simulink library "srx_platform"  (Simulink 8.2)
settings: Solver=ode1  StartTime=0.0  StopTime=Inf  FixedStep=0.001  RelTol=1e-3
PostLoadFcn:
  | , if any(exist('dsrtsu_mdlpostloadfcn', 'file') == [2, 3, 6]), try dsrtsu_mdlpostloadfcn('Execute', bdroot); catch fprintf('Error in PostLoadFcn (dsrtsu_mdlpostloadfcn) for model "%s":\n %s\n', bdroot, lasterr); end, end,
libraries: rtican x23, rtiethernetudplib x4, srx_initialize x4, rtiflashlib x2, topr5_adapter x1
(part 2 of 6)

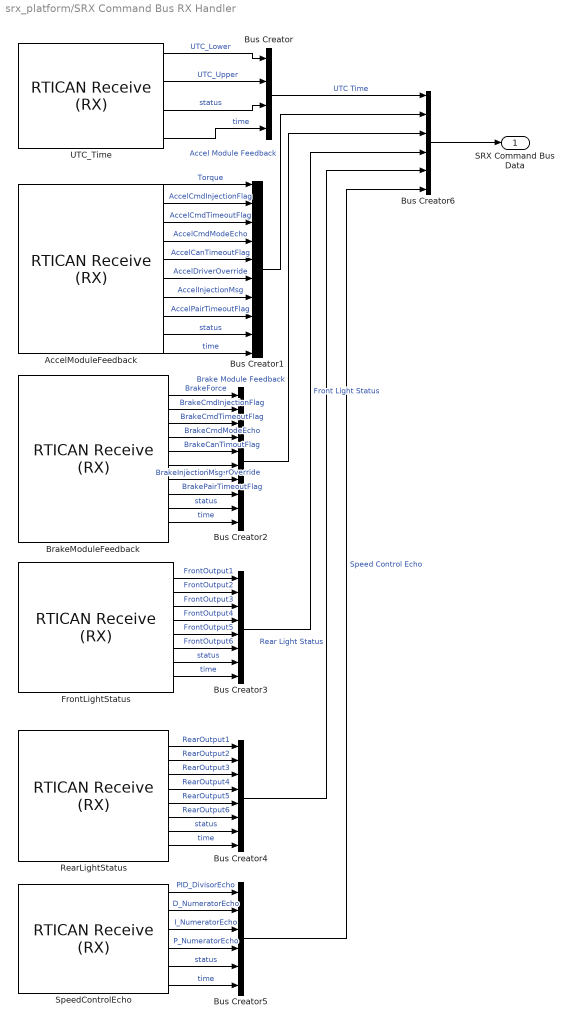
== system srx_platform/SRX Command Bus RX Handler ==
  AccelModuleFeedback : rtican/RTICAN Receive (RX)   Reserved1=[]  Reserved2=[]  Reserved3=[]  Reserved4=[]  SfcnMessage=[]  Msg_Struct=[]  BoardTypeNo=[]  BoardNo=[]  ChannelNo=[]  Parameters=[]  DialogFcn=[]  UnitName=[]  Revision=[]  UnitValues=[]  DSProperties=struct('RTI',struct('Version',uint32(5),'BlockType',struct('isSLSource',uint8(1),'isSLSink',uint8(1),'isHWSource',uint8(0),'isHWSink',uint8(0),'isSetup',uint8(0),'isInline',uint8(1),'isNonInline',uint8(0),'isInterrupt',uint8(0),'isChannelwise',uint8(0)),'IOBoardType','RTICAN','UnitType','MESSAGE','Identifier','RX','DialogType','MSVC','BlockSet','RTICAN','SlaveProcessor','CAN'))  RTIBlockInterface=struct('OutputPortsWidth',int32([1 1 1 1 1 1 1 1 1 1]),'OutputPortsActive',[1 1 1 1 1 1 1 1 1 1],'OutputPortsName',{{'Torque','AccelCmdInjectionFlag','AccelCmdTimeoutFlag','AccelCmdModeEcho','AccelCanTimeoutFlag','AccelDriverOverride','AccelInjectionMsg','AccelPairTimeoutFlag',['RX status'],['RX time']}},'OutputPortsDataType',{{'SS_UINT32','SS_BOOLEAN','SS_BOOLEAN','SS_UINT8','SS_BOOLEAN','SS_BOOLEAN','SS_BOOLEAN','SS_BOOLEAN','SS_DOUBLE','SS_DOUBLE'}},'OutputPortsLabel',{{'Torque','AccelCmdInjectionFlag','AccelCmdTimeoutFlag','AccelCmdModeEcho','AccelCanTimeoutFlag','AccelDriverOverride','AccelInjectionMsg','AccelPairTimeoutFlag','',''}},'OutputPortsLabelMode','ON','InputPortsWidth',int32(0),'InputPortsActive',0,'DialogFcn','rtican_message_interface_gui','BlockDisplay',{{'','center'}},'IconTransparency','on','ParameterTunableNames',{{}},'InitLevel',3,'BlockName',struct('Token',{{'AccelModuleFeedback'}}),'SampleTime',{{-1}},'TriggerPort',{{'none'}},'EnablePort',{{'none'}})  RTIBlockParameters=struct('BoardTypeNo',{{1,'OFF',[]}},'BoardNo',{{2,'ON',[1 16]}},'ChannelNo',{{1,'ON',[1 2]}},'Parameters',{{struct('DataFileSupport',struct('DataFileSelectedMaster',1,'DataFileSelectedLocal',1,'DataFileName','c:\users\leidos\development\carmaplatform\microautobox\src\data_files\srx_command.dbc|','DataFileDate',['17-Aug-2015 10:52:13'],'SelectedFile','..\data_files\srx_command.dbc','InterfaceFcn','rtican_dbc_file_parser'),'Options',struct('StatusSelected',1,'TimeSelected',1,'DeltaTimeSelected',0,'BytePortSelected',0,'MessageLengthSelected',0,'TriggerPort',struct('Selected',0,'TriggerType',0),'UserCoding',struct('Selected',0,'InterfaceFile','UserDecodingFile','FcnName','UserDecodeFcn','InportSelected',0,'InportWidth',1,'OutportSelected',0,'OutportWidth',1),'EnablePortSelected',0,'SignalOnPortnameSelected',1,'UseRXService',1),'Message',struct('MsgOnBlocknameSelected',1,'MsgName','AccelModuleFeedback','MsgIdFormat',0,'MsgId',416,'MsgLength',4,'NumSignals',8,'SampleTime',-1,'Signal',struct('SgnName',{'Torque','AccelCmdInjectionFlag','AccelCmdTimeoutFlag','AccelCmdModeEcho','AccelCanTimeoutFlag','AccelDriverOverride','AccelInjectionMsg','AccelPairTimeoutFlag'},'SgnStartBit',{0,24,25,26,28,29,30,31},'SgnLength',{24,1,1,2,1,1,1,1},'ByteLayout',{2,2,2,2,2,2,2,2},'Factor',{1,1,1,1,1,1,1,1},'Offset',{0,0,0,0,0,0,0,0},'SgnComment',{'','','','','','','',''},'SgnUnit',{'','','','','','','',''},'Min',{0,0,0,0,0,0,0,0},'Max',{0,0,0,0,0,0,0,0},'SgnType',{0,0,0,0,0,0,0,0},'SLDataType',{'SS_UINT32','SS_BOOLEAN','SS_BOOLEAN','SS_UINT8','SS_BOOLEAN','SS_BOOLEAN','SS_BOOLEAN','SS_BOOLEAN'},'DataType',{0,0,0,0,0,0,0,0},'ModeValue',{-1,-1,-1,-1,-1,-1,-1,-1}),'MsgIdNumFormat',0,'MsgComment',{{''}}),'Version',1.2,'general',struct('isFromLib',0)),'OFF',[]}},'GroupId',{{struct('Group',{{'RTICAN'}},'No',3,'Behavior',{{'NAMECHANGE'}},'BlockType',{{'SINK'}},'NameChangeFlag',0),'OFF',[]}},'SFcnRTICANMessage',{{struct('MsgType','RX','SFcnPortType','Scalar','MsgName','AccelModuleFeedback','MsgIdFormat','STD','MsgId',416,'MsgLength',4,'NumSignals',8,'SampleTime',-1,'Signal',struct('SgnName',{'Torque','AccelCmdInjectionFlag','AccelCmdTimeoutFlag','AccelCmdModeEcho','AccelCanTimeoutFlag','AccelDriverOverride','AccelInjectionMsg','AccelPairTimeoutFlag'},'SgnStartBit',{0,24,25,26,28,29,30,31},'SgnLength',{24,1,1,2,1,1,1,1},'ByteLayout',{['motorola back.'],['motorola back.'],['motorola back.'],['motorola back.'],['motorola back.'],['motorola back.'],['motorola back.'],['motorola back.']},'Factor',{1,1,1,1,1,1,1,1},'Offset',{0,0,0,0,0,0,0,0},'SgnType',{'standard','standard','standard','standard','standard','standard','standard','standard'},'SLDataType',{'SS_UINT32','SS_BOOLEAN','SS_BOOLEAN','SS_UINT8','SS_BOOLEAN','SS_BOOLEAN','SS_BOOLEAN','SS_BOOLEAN'},'DataType',{['unsigned int'],['unsigned int'],['unsigned int'],['unsigned int'],['unsigned int'],['unsigned int'],['unsigned int'],['unsigned int']},'ModeValue',{-1,-1,-1,-1,-1,-1,-1,-1}),'StatusSelected','yes','TimeSelected','yes','DeltaTimeSelected','no','BytePortSelected','no','MessageLengthSelected','no','TriggerPort',struct('Selected','no','TriggerType',0),'UserCoding',struct('Selected','no','InterfaceFile','UserDecodingFile','FcnName','UserDecodeFcn','InportSelected','no','InportWidth',1,'OutportSelected','no','OutportWidth',1),'EnablePortSelected','no','UseRXService','yes','BoardType','DS1','BoardNo',2,'ControllerNo',1),'OFF',[]}},'TLCFileName',{{'rtican_rx_message','OFF',[]}})  RTISFcnParameters=struct('SFcnRTICANMessage','struct','TLCFileName','char')  RTIBlockParaDefault=struct('BoardTypeNo',4302,'BoardNo',1,'ChannelNo',1,'Parameters',struct('DataFileSupport',struct('DataFileSelectedMaster',0,'DataFileSelectedLocal',0,'DataFileName','','DataFileDate','','SelectedFile',['<no file selected>']),'Options',struct('StatusSelected',1,'TimeSelected',1,'DeltaTimeSelected',1,'BytePortSelected',0,'MessageLengthSelected',0,'TriggerPort',struct('Selected',0,'TriggerType','rising'),'UserCoding',struct('Selected',0,'InterfaceFile','UserDecodingFile','FcnName','UserDecodeFcn','InportSelected',0,'InportWidth',1,'OutportSelected',0,'OutportWidth',1),'EnablePortSelected',0,'SignalOnPortnameSelected',1,'UseRXService',0),'Message',struct('MsgOnBlocknameSelected',0,'MsgName',['RX Message'],'MsgIdFormat',0,'MsgId',100,'MsgLength',8,'NumSignals',1,'SampleTime',-1,'Signal',struct('SgnName',['RX signal'],'SgnStartBit',0,'SgnLength',8,'SgnType',0,'ModeValue',-1,'DataType',0,'SLDataType','SS_DOUBLE','ByteLayout',0,'Factor',1,'Offset',0,'Min',0,'Max',255,'SgnComment',{{}},'SgnUnit',''),'MsgIdNumFormat',0,'MsgComment',{{''}}),'Version',1.2,'general',struct('isFromLib',1)),'GroupId',struct('Group',{{'RTICAN'}},'No',1,'Behavior',{{'NAMECHANGE'}},'BlockType',{{'SINK'}},'NameChangeFlag',0),'SFcnRTICANMessage',struct('MsgType','RX','MsgName',['RX Message'],'MsgIdFormat','STD','MsgId',100,'MsgLength',8,'NumSignals',1,'SampleTime',-1,'Signal',struct('SgnName',['RX signal'],'SgnStartBit',0,'SgnLength',8,'SgnType','standard','ModeValue',-1,'DataType',['unsigned int'],'ByteLayout',['little endian'],'SLDataType','SS_DOUBLE','Factor',1,'Offset',0),'StatusSelected','yes','TimeSelected','yes','DeltaTimeSelected','yes','BytePortSelected','no','MessageLengthSelected','no','EnablePortSelected','no','UserCoding',struct('Selected','no','InterfaceFile','UserDecodingFile','FcnName','UserDecodeFcn','InportSelected','no','InportWidth',1,'OutportSelected','no','OutportWidth',1),'TriggerPort',struct('Selected','no','TriggerType','rising'),'UseRXService','no','BoardType','DS4302','BoardNo',1,'ControllerNo',1,'SFcnPortType','Scalar'),'TLCFileName','rtican_rx_message')
      settings: AttributesFormatString=Group Id: RTICAN3\n
  BrakeModuleFeedback : rtican/RTICAN Receive (RX)   Reserved1=[]  Reserved2=[]  Reserved3=[]  Reserved4=[]  SfcnMessage=[]  Msg_Struct=[]  BoardTypeNo=[]  BoardNo=[]  ChannelNo=[]  Parameters=[]  DialogFcn=[]  UnitName=[]  Revision=[]  UnitValues=[]  DSProperties=struct('RTI',struct('Version',uint32(5),'BlockType',struct('isSLSource',uint8(1),'isSLSink',uint8(1),'isHWSource',uint8(0),'isHWSink',uint8(0),'isSetup',uint8(0),'isInline',uint8(1),'isNonInline',uint8(0),'isInterrupt',uint8(0),'isChannelwise',uint8(0)),'IOBoardType','RTICAN','UnitType','MESSAGE','Identifier','RX','DialogType','MSVC','BlockSet','RTICAN','SlaveProcessor','CAN'))  RTIBlockInterface=struct('OutputPortsWidth',int32([1 1 1 1 1 1 1 1 1 1]),'OutputPortsActive',[1 1 1 1 1 1 1 1 1 1],'OutputPortsName',{{'BrakeForce','BrakeCmdInjectionFlag','BrakeCmdTimeoutFlag','BrakeCmdModeEcho','BrakeCanTimoutFlag','BrakeDriverOverride','BrakeInjectionMsg','BrakePairTimeoutFlag',['RX status'],['RX time']}},'OutputPortsDataType',{{'SS_DOUBLE','SS_BOOLEAN','SS_BOOLEAN','SS_UINT8','SS_BOOLEAN','SS_BOOLEAN','SS_BOOLEAN','SS_BOOLEAN','SS_DOUBLE','SS_DOUBLE'}},'OutputPortsLabel',{{'BrakeForce','BrakeCmdInjectionFlag','BrakeCmdTimeoutFlag','BrakeCmdModeEcho','BrakeCanTimoutFlag','BrakeDriverOverride','BrakeInjectionMsg','BrakePairTimeoutFlag','',''}},'OutputPortsLabelMode','ON','InputPortsWidth',int32(0),'InputPortsActive',0,'DialogFcn','rtican_message_interface_gui','BlockDisplay',{{'','center'}},'IconTransparency','on','ParameterTunableNames',{{}},'InitLevel',3,'BlockName',struct('Token',{{'BrakeModuleFeedback'}}),'SampleTime',{{-1}},'TriggerPort',{{'none'}},'EnablePort',{{'none'}})  RTIBlockParameters=struct('BoardTypeNo',{{1,'OFF',[]}},'BoardNo',{{2,'ON',[1 16]}},'ChannelNo',{{1,'ON',[1 2]}},'Parameters',{{struct('DataFileSupport',struct('DataFileSelectedMaster',1,'DataFileSelectedLocal',1,'DataFileName','c:\users\leidos\development\carmaplatform\microautobox\src\data_files\srx_command.dbc|','DataFileDate',['17-Aug-2015 10:52:13'],'SelectedFile','..\data_files\srx_command.dbc','InterfaceFcn','rtican_dbc_file_parser'),'Options',struct('StatusSelected',1,'TimeSelected',1,'DeltaTimeSelected',0,'BytePortSelected',0,'MessageLengthSelected',0,'TriggerPort',struct('Selected',0,'TriggerType',0),'UserCoding',struct('Selected',0,'InterfaceFile','UserDecodingFile','FcnName','UserDecodeFcn','InportSelected',0,'InportWidth',1,'OutportSelected',0,'OutportWidth',1),'EnablePortSelected',0,'SignalOnPortnameSelected',1,'UseRXService',1),'Message',struct('MsgOnBlocknameSelected',1,'MsgName','BrakeModuleFeedback','MsgIdFormat',0,'MsgId',432,'MsgLength',3,'NumSignals',8,'SampleTime',-1,'Signal',struct('SgnName',{'BrakeForce','BrakeCmdInjectionFlag','BrakeCmdTimeoutFlag','BrakeCmdModeEcho','BrakeCanTimoutFlag','BrakeDriverOverride','BrakeInjectionMsg','BrakePairTimeoutFlag'},'SgnStartBit',{0,16,17,18,20,21,22,23},'SgnLength',{12,1,1,2,1,1,1,1},'ByteLayout',{2,2,2,2,2,2,2,2},'Factor',{0.01,1,1,1,1,1,1,1},'Offset',{-20.48,0,0,0,0,0,0,0},'SgnComment',{'','','','','','','',''},'SgnUnit',{'','','','','','','',''},'Min',{0,0,0,0,0,0,0,0},'Max',{0,0,0,0,0,0,0,0},'SgnType',{0,0,0,0,0,0,0,0},'SLDataType',{'SS_DOUBLE','SS_BOOLEAN','SS_BOOLEAN','SS_UINT8','SS_BOOLEAN','SS_BOOLEAN','SS_BOOLEAN','SS_BOOLEAN'},'DataType',{0,0,0,0,0,0,0,0},'ModeValue',{-1,-1,-1,-1,-1,-1,-1,-1}),'MsgIdNumFormat',0,'MsgComment',{{''}}),'Version',1.2,'general',struct('isFromLib',0)),'OFF',[]}},'GroupId',{{struct('Group',{{'RTICAN'}},'No',3,'Behavior',{{'NAMECHANGE'}},'BlockType',{{'SINK'}},'NameChangeFlag',0),'OFF',[]}},'SFcnRTICANMessage',{{struct('MsgType','RX','SFcnPortType','Scalar','MsgName','BrakeModuleFeedback','MsgIdFormat','STD','MsgId',432,'MsgLength',3,'NumSignals',8,'SampleTime',-1,'Signal',struct('SgnName',{'BrakeForce','BrakeCmdInjectionFlag','BrakeCmdTimeoutFlag','BrakeCmdModeEcho','BrakeCanTimoutFlag','BrakeDriverOverride','BrakeInjectionMsg','BrakePairTimeoutFlag'},'SgnStartBit',{0,16,17,18,20,21,22,23},'SgnLength',{12,1,1,2,1,1,1,1},'ByteLayout',{['motorola back.'],['motorola back.'],['motorola back.'],['motorola back.'],['motorola back.'],['motorola back.'],['motorola back.'],['motorola back.']},'Factor',{0.01,1,1,1,1,1,1,1},'Offset',{-20.48,0,0,0,0,0,0,0},'SgnType',{'standard','standard','standard','standard','standard','standard','standard','standard'},'SLDataType',{'SS_DOUBLE','SS_BOOLEAN','SS_BOOLEAN','SS_UINT8','SS_BOOLEAN','SS_BOOLEAN','SS_BOOLEAN','SS_BOOLEAN'},'DataType',{['unsigned int'],['unsigned int'],['unsigned int'],['unsigned int'],['unsigned int'],['unsigned int'],['unsigned int'],['unsigned int']},'ModeValue',{-1,-1,-1,-1,-1,-1,-1,-1}),'StatusSelected','yes','TimeSelected','yes','DeltaTimeSelected','no','BytePortSelected','no','MessageLengthSelected','no','TriggerPort',struct('Selected','no','TriggerType',0),'UserCoding',struct('Selected','no','InterfaceFile','UserDecodingFile','FcnName','UserDecodeFcn','InportSelected','no','InportWidth',1,'OutportSelected','no','OutportWidth',1),'EnablePortSelected','no','UseRXService','yes','BoardType','DS1','BoardNo',2,'ControllerNo',1),'OFF',[]}},'TLCFileName',{{'rtican_rx_message','OFF',[]}})  RTISFcnParameters=struct('SFcnRTICANMessage','struct','TLCFileName','char')  RTIBlockParaDefault=struct('BoardTypeNo',4302,'BoardNo',1,'ChannelNo',1,'Parameters',struct('DataFileSupport',struct('DataFileSelectedMaster',0,'DataFileSelectedLocal',0,'DataFileName','','DataFileDate','','SelectedFile',['<no file selected>']),'Options',struct('StatusSelected',1,'TimeSelected',1,'DeltaTimeSelected',1,'BytePortSelected',0,'MessageLengthSelected',0,'TriggerPort',struct('Selected',0,'TriggerType','rising'),'UserCoding',struct('Selected',0,'InterfaceFile','UserDecodingFile','FcnName','UserDecodeFcn','InportSelected',0,'InportWidth',1,'OutportSelected',0,'OutportWidth',1),'EnablePortSelected',0,'SignalOnPortnameSelected',1,'UseRXService',0),'Message',struct('MsgOnBlocknameSelected',0,'MsgName',['RX Message'],'MsgIdFormat',0,'MsgId',100,'MsgLength',8,'NumSignals',1,'SampleTime',-1,'Signal',struct('SgnName',['RX signal'],'SgnStartBit',0,'SgnLength',8,'SgnType',0,'ModeValue',-1,'DataType',0,'SLDataType','SS_DOUBLE','ByteLayout',0,'Factor',1,'Offset',0,'Min',0,'Max',255,'SgnComment',{{}},'SgnUnit',''),'MsgIdNumFormat',0,'MsgComment',{{''}}),'Version',1.2,'general',struct('isFromLib',1)),'GroupId',struct('Group',{{'RTICAN'}},'No',1,'Behavior',{{'NAMECHANGE'}},'BlockType',{{'SINK'}},'NameChangeFlag',0),'SFcnRTICANMessage',struct('MsgType','RX','MsgName',['RX Message'],'MsgIdFormat','STD','MsgId',100,'MsgLength',8,'NumSignals',1,'SampleTime',-1,'Signal',struct('SgnName',['RX signal'],'SgnStartBit',0,'SgnLength',8,'SgnType','standard','ModeValue',-1,'DataType',['unsigned int'],'ByteLayout',['little endian'],'SLDataType','SS_DOUBLE','Factor',1,'Offset',0),'StatusSelected','yes','TimeSelected','yes','DeltaTimeSelected','yes','BytePortSelected','no','MessageLengthSelected','no','EnablePortSelected','no','UserCoding',struct('Selected','no','InterfaceFile','UserDecodingFile','FcnName','UserDecodeFcn','InportSelected','no','InportWidth',1,'OutportSelected','no','OutportWidth',1),'TriggerPort',struct('Selected','no','TriggerType','rising'),'UseRXService','no','BoardType','DS4302','BoardNo',1,'ControllerNo',1,'SFcnPortType','Scalar'),'TLCFileName','rtican_rx_message')
      settings: AttributesFormatString=Group Id: RTICAN3\n
  Bus Creator : BusCreator
  Bus Creator1 : BusCreator  Inputs=10
  Bus Creator2 : BusCreator  Inputs=10
  Bus Creator3 : BusCreator  Inputs=8
  Bus Creator4 : BusCreator  Inputs=8
  Bus Creator5 : BusCreator  Inputs=6
  Bus Creator6 : BusCreator  Inputs=6
  FrontLightStatus : rtican/RTICAN Receive (RX)   Reserved1=[]  Reserved2=[]  Reserved3=[]  Reserved4=[]  SfcnMessage=[]  Msg_Struct=[]  BoardTypeNo=[]  BoardNo=[]  ChannelNo=[]  Parameters=[]  DialogFcn=[]  UnitName=[]  Revision=[]  UnitValues=[]  DSProperties=struct('RTI',struct('Version',uint32(5),'BlockType',struct('isSLSource',uint8(1),'isSLSink',uint8(1),'isHWSource',uint8(0),'isHWSink',uint8(0),'isSetup',uint8(0),'isInline',uint8(1),'isNonInline',uint8(0),'isInterrupt',uint8(0),'isChannelwise',uint8(0)),'IOBoardType','RTICAN','UnitType','MESSAGE','Identifier','RX','DialogType','MSVC','BlockSet','RTICAN','SlaveProcessor','CAN'))  RTIBlockInterface=struct('OutputPortsWidth',int32([1 1 1 1 1 1 1 1]),'OutputPortsActive',[1 1 1 1 1 1 1 1],'OutputPortsName',{{'FrontOutput1','FrontOutput2','FrontOutput3','FrontOutput4','FrontOutput5','FrontOutput6',['RX status'],['RX time']}},'OutputPortsDataType',{{'SS_BOOLEAN','SS_BOOLEAN','SS_BOOLEAN','SS_BOOLEAN','SS_BOOLEAN','SS_BOOLEAN','SS_DOUBLE','SS_DOUBLE'}},'OutputPortsLabel',{{'FrontOutput1','FrontOutput2','FrontOutput3','FrontOutput4','FrontOutput5','FrontOutput6','',''}},'OutputPortsLabelMode','ON','InputPortsWidth',int32(0),'InputPortsActive',0,'DialogFcn','rtican_message_interface_gui','BlockDisplay',{{'','center'}},'IconTransparency','on','ParameterTunableNames',{{}},'InitLevel',3,'BlockName',struct('Token',{{'FrontLightStatus'}}),'SampleTime',{{-1}},'TriggerPort',{{'none'}},'EnablePort',{{'none'}})  RTIBlockParameters=struct('BoardTypeNo',{{1,'OFF',[]}},'BoardNo',{{2,'ON',[1 16]}},'ChannelNo',{{1,'ON',[1 2]}},'Parameters',{{struct('DataFileSupport',struct('DataFileSelectedMaster',1,'DataFileSelectedLocal',1,'DataFileName','c:\users\leidos\development\carmaplatform\microautobox\src\data_files\srx_command.dbc|','DataFileDate',['17-Aug-2015 10:52:13'],'SelectedFile','..\data_files\srx_command.dbc','InterfaceFcn','rtican_dbc_file_parser'),'Options',struct('StatusSelected',1,'TimeSelected',1,'DeltaTimeSelected',0,'BytePortSelected',0,'MessageLengthSelected',0,'TriggerPort',struct('Selected',0,'TriggerType',0),'UserCoding',struct('Selected',0,'InterfaceFile','UserDecodingFile','FcnName','UserDecodeFcn','InportSelected',0,'InportWidth',1,'OutportSelected',0,'OutportWidth',1),'EnablePortSelected',0,'SignalOnPortnameSelected',1,'UseRXService',1),'Message',struct('MsgOnBlocknameSelected',1,'MsgName','FrontLightStatus','MsgIdFormat',0,'MsgId',275,'MsgLength',1,'NumSignals',6,'SampleTime',-1,'Signal',struct('SgnName',{'FrontOutput1','FrontOutput2','FrontOutput3','FrontOutput4','FrontOutput5','FrontOutput6'},'SgnStartBit',{0,1,2,3,4,5},'SgnLength',{1,1,1,1,1,1},'ByteLayout',{2,2,2,2,2,2},'Factor',{1,1,1,1,1,1},'Offset',{0,0,0,0,0,0},'SgnComment',{['Unassigned Output'],['Left Arrow'],['Right Arrow'],'Takedown','Flash',['Unassigned Output']},'SgnUnit',{'','','','','',''},'Min',{0,0,0,0,0,0},'Max',{0,0,0,0,0,0},'SgnType',{0,0,0,0,0,0},'SLDataType',{'SS_BOOLEAN','SS_BOOLEAN','SS_BOOLEAN','SS_BOOLEAN','SS_BOOLEAN','SS_BOOLEAN'},'DataType',{0,0,0,0,0,0},'ModeValue',{-1,-1,-1,-1,-1,-1}),'MsgIdNumFormat',0,'MsgComment',{{''}}),'Version',1.2,'general',struct('isFromLib',0)),'OFF',[]}},'GroupId',{{struct('Group',{{'RTICAN'}},'No',3,'Behavior',{{'NAMECHANGE'}},'BlockType',{{'SINK'}},'NameChangeFlag',0),'OFF',[]}},'SFcnRTICANMessage',{{struct('MsgType','RX','SFcnPortType','Scalar','MsgName','FrontLightStatus','MsgIdFormat','STD','MsgId',275,'MsgLength',1,'NumSignals',6,'SampleTime',-1,'Signal',struct('SgnName',{'FrontOutput1','FrontOutput2','FrontOutput3','FrontOutput4','FrontOutput5','FrontOutput6'},'SgnStartBit',{0,1,2,3,4,5},'SgnLength',{1,1,1,1,1,1},'ByteLayout',{['motorola back.'],['motorola back.'],['motorola back.'],['motorola back.'],['motorola back.'],['motorola back.']},'Factor',{1,1,1,1,1,1},'Offset',{0,0,0,0,0,0},'SgnType',{'standard','standard','standard','standard','standard','standard'},'SLDataType',{'SS_BOOLEAN','SS_BOOLEAN','SS_BOOLEAN','SS_BOOLEAN','SS_BOOLEAN','SS_BOOLEAN'},'DataType',{['unsigned int'],['unsigned int'],['unsigned int'],['unsigned int'],['unsigned int'],['unsigned int']},'ModeValue',{-1,-1,-1,-1,-1,-1}),'StatusSelected','yes','TimeSelected','yes','DeltaTimeSelected','no','BytePortSelected','no','MessageLengthSelected','no','TriggerPort',struct('Selected','no','TriggerType',0),'UserCoding',struct('Selected','no','InterfaceFile','UserDecodingFile','FcnName','UserDecodeFcn','InportSelected','no','InportWidth',1,'OutportSelected','no','OutportWidth',1),'EnablePortSelected','no','UseRXService','yes','BoardType','DS1','BoardNo',2,'ControllerNo',1),'OFF',[]}},'TLCFileName',{{'rtican_rx_message','OFF',[]}})  RTISFcnParameters=struct('SFcnRTICANMessage','struct','TLCFileName','char')  RTIBlockParaDefault=struct('BoardTypeNo',4302,'BoardNo',1,'ChannelNo',1,'Parameters',struct('DataFileSupport',struct('DataFileSelectedMaster',0,'DataFileSelectedLocal',0,'DataFileName','','DataFileDate','','SelectedFile',['<no file selected>']),'Options',struct('StatusSelected',1,'TimeSelected',1,'DeltaTimeSelected',1,'BytePortSelected',0,'MessageLengthSelected',0,'TriggerPort',struct('Selected',0,'TriggerType','rising'),'UserCoding',struct('Selected',0,'InterfaceFile','UserDecodingFile','FcnName','UserDecodeFcn','InportSelected',0,'InportWidth',1,'OutportSelected',0,'OutportWidth',1),'EnablePortSelected',0,'SignalOnPortnameSelected',1,'UseRXService',0),'Message',struct('MsgOnBlocknameSelected',0,'MsgName',['RX Message'],'MsgIdFormat',0,'MsgId',100,'MsgLength',8,'NumSignals',1,'SampleTime',-1,'Signal',struct('SgnName',['RX signal'],'SgnStartBit',0,'SgnLength',8,'SgnType',0,'ModeValue',-1,'DataType',0,'SLDataType','SS_DOUBLE','ByteLayout',0,'Factor',1,'Offset',0,'Min',0,'Max',255,'SgnComment',{{}},'SgnUnit',''),'MsgIdNumFormat',0,'MsgComment',{{''}}),'Version',1.2,'general',struct('isFromLib',1)),'GroupId',struct('Group',{{'RTICAN'}},'No',1,'Behavior',{{'NAMECHANGE'}},'BlockType',{{'SINK'}},'NameChangeFlag',0),'SFcnRTICANMessage',struct('MsgType','RX','MsgName',['RX Message'],'MsgIdFormat','STD','MsgId',100,'MsgLength',8,'NumSignals',1,'SampleTime',-1,'Signal',struct('SgnName',['RX signal'],'SgnStartBit',0,'SgnLength',8,'SgnType','standard','ModeValue',-1,'DataType',['unsigned int'],'ByteLayout',['little endian'],'SLDataType','SS_DOUBLE','Factor',1,'Offset',0),'StatusSelected','yes','TimeSelected','yes','DeltaTimeSelected','yes','BytePortSelected','no','MessageLengthSelected','no','EnablePortSelected','no','UserCoding',struct('Selected','no','InterfaceFile','UserDecodingFile','FcnName','UserDecodeFcn','InportSelected','no','InportWidth',1,'OutportSelected','no','OutportWidth',1),'TriggerPort',struct('Selected','no','TriggerType','rising'),'UseRXService','no','BoardType','DS4302','BoardNo',1,'ControllerNo',1,'SFcnPortType','Scalar'),'TLCFileName','rtican_rx_message')
      settings: AttributesFormatString=Group Id: RTICAN3\n
  RearLightStatus : rtican/RTICAN Receive (RX)   Reserved1=[]  Reserved2=[]  Reserved3=[]  Reserved4=[]  SfcnMessage=[]  Msg_Struct=[]  BoardTypeNo=[]  BoardNo=[]  ChannelNo=[]  Parameters=[]  DialogFcn=[]  UnitName=[]  Revision=[]  UnitValues=[]  DSProperties=struct('RTI',struct('Version',uint32(5),'BlockType',struct('isSLSource',uint8(1),'isSLSink',uint8(1),'isHWSource',uint8(0),'isHWSink',uint8(0),'isSetup',uint8(0),'isInline',uint8(1),'isNonInline',uint8(0),'isInterrupt',uint8(0),'isChannelwise',uint8(0)),'IOBoardType','RTICAN','UnitType','MESSAGE','Identifier','RX','DialogType','MSVC','BlockSet','RTICAN','SlaveProcessor','CAN'))  RTIBlockInterface=struct('OutputPortsWidth',int32([1 1 1 1 1 1 1 1]),'OutputPortsActive',[1 1 1 1 1 1 1 1],'OutputPortsName',{{'RearOutput1','RearOutput2','RearOutput3','RearOutput4','RearOutput5','RearOutput6',['RX status'],['RX time']}},'OutputPortsDataType',{{'SS_BOOLEAN','SS_BOOLEAN','SS_BOOLEAN','SS_BOOLEAN','SS_BOOLEAN','SS_BOOLEAN','SS_DOUBLE','SS_DOUBLE'}},'OutputPortsLabel',{{'RearOutput1','RearOutput2','RearOutput3','RearOutput4','RearOutput5','RearOutput6','',''}},'OutputPortsLabelMode','ON','InputPortsWidth',int32(0),'InputPortsActive',0,'DialogFcn','rtican_message_interface_gui','BlockDisplay',{{'','center'}},'IconTransparency','on','ParameterTunableNames',{{}},'InitLevel',3,'BlockName',struct('Token',{{'RearLightStatus'}}),'SampleTime',{{-1}},'TriggerPort',{{'none'}},'EnablePort',{{'none'}})  RTIBlockParameters=struct('BoardTypeNo',{{1,'OFF',[]}},'BoardNo',{{2,'ON',[1 16]}},'ChannelNo',{{1,'ON',[1 2]}},'Parameters',{{struct('DataFileSupport',struct('DataFileSelectedMaster',1,'DataFileSelectedLocal',1,'DataFileName','c:\users\leidos\development\carmaplatform\microautobox\src\data_files\srx_command.dbc|','DataFileDate',['17-Aug-2015 10:52:13'],'SelectedFile','..\data_files\srx_command.dbc','InterfaceFcn','rtican_dbc_file_parser'),'Options',struct('StatusSelected',1,'TimeSelected',1,'DeltaTimeSelected',0,'BytePortSelected',0,'MessageLengthSelected',0,'TriggerPort',struct('Selected',0,'TriggerType',0),'UserCoding',struct('Selected',0,'InterfaceFile','UserDecodingFile','FcnName','UserDecodeFcn','InportSelected',0,'InportWidth',1,'OutportSelected',0,'OutportWidth',1),'EnablePortSelected',0,'SignalOnPortnameSelected',1,'UseRXService',1),'Message',struct('MsgOnBlocknameSelected',1,'MsgName','RearLightStatus','MsgIdFormat',0,'MsgId',276,'MsgLength',1,'NumSignals',6,'SampleTime',-1,'Signal',struct('SgnName',{'RearOutput1','RearOutput2','RearOutput3','RearOutput4','RearOutput5','RearOutput6'},'SgnStartBit',{0,1,2,3,4,5},'SgnLength',{1,1,1,1,1,1},'ByteLayout',{2,2,2,2,2,2},'Factor',{1,1,1,1,1,1},'Offset',{0,0,0,0,0,0},'SgnComment',{['Unassigned Output'],['Left Arrow'],['Right Arrow'],'Takedown','Flash',['Unassigned Output']},'SgnUnit',{'','','','','',''},'Min',{0,0,0,0,0,0},'Max',{0,0,0,0,0,0},'SgnType',{0,0,0,0,0,0},'SLDataType',{'SS_BOOLEAN','SS_BOOLEAN','SS_BOOLEAN','SS_BOOLEAN','SS_BOOLEAN','SS_BOOLEAN'},'DataType',{0,0,0,0,0,0},'ModeValue',{-1,-1,-1,-1,-1,-1}),'MsgIdNumFormat',0,'MsgComment',{{''}}),'Version',1.2,'general',struct('isFromLib',0)),'OFF',[]}},'GroupId',{{struct('Group',{{'RTICAN'}},'No',3,'Behavior',{{'NAMECHANGE'}},'BlockType',{{'SINK'}},'NameChangeFlag',0),'OFF',[]}},'SFcnRTICANMessage',{{struct('MsgType','RX','SFcnPortType','Scalar','MsgName','RearLightStatus','MsgIdFormat','STD','MsgId',276,'MsgLength',1,'NumSignals',6,'SampleTime',-1,'Signal',struct('SgnName',{'RearOutput1','RearOutput2','RearOutput3','RearOutput4','RearOutput5','RearOutput6'},'SgnStartBit',{0,1,2,3,4,5},'SgnLength',{1,1,1,1,1,1},'ByteLayout',{['motorola back.'],['motorola back.'],['motorola back.'],['motorola back.'],['motorola back.'],['motorola back.']},'Factor',{1,1,1,1,1,1},'Offset',{0,0,0,0,0,0},'SgnType',{'standard','standard','standard','standard','standard','standard'},'SLDataType',{'SS_BOOLEAN','SS_BOOLEAN','SS_BOOLEAN','SS_BOOLEAN','SS_BOOLEAN','SS_BOOLEAN'},'DataType',{['unsigned int'],['unsigned int'],['unsigned int'],['unsigned int'],['unsigned int'],['unsigned int']},'ModeValue',{-1,-1,-1,-1,-1,-1}),'StatusSelected','yes','TimeSelected','yes','DeltaTimeSelected','no','BytePortSelected','no','MessageLengthSelected','no','TriggerPort',struct('Selected','no','TriggerType',0),'UserCoding',struct('Selected','no','InterfaceFile','UserDecodingFile','FcnName','UserDecodeFcn','InportSelected','no','InportWidth',1,'OutportSelected','no','OutportWidth',1),'EnablePortSelected','no','UseRXService','yes','BoardType','DS1','BoardNo',2,'ControllerNo',1),'OFF',[]}},'TLCFileName',{{'rtican_rx_message','OFF',[]}})  RTISFcnParameters=struct('SFcnRTICANMessage','struct','TLCFileName','char')  RTIBlockParaDefault=struct('BoardTypeNo',4302,'BoardNo',1,'ChannelNo',1,'Parameters',struct('DataFileSupport',struct('DataFileSelectedMaster',0,'DataFileSelectedLocal',0,'DataFileName','','DataFileDate','','SelectedFile',['<no file selected>']),'Options',struct('StatusSelected',1,'TimeSelected',1,'DeltaTimeSelected',1,'BytePortSelected',0,'MessageLengthSelected',0,'TriggerPort',struct('Selected',0,'TriggerType','rising'),'UserCoding',struct('Selected',0,'InterfaceFile','UserDecodingFile','FcnName','UserDecodeFcn','InportSelected',0,'InportWidth',1,'OutportSelected',0,'OutportWidth',1),'EnablePortSelected',0,'SignalOnPortnameSelected',1,'UseRXService',0),'Message',struct('MsgOnBlocknameSelected',0,'MsgName',['RX Message'],'MsgIdFormat',0,'MsgId',100,'MsgLength',8,'NumSignals',1,'SampleTime',-1,'Signal',struct('SgnName',['RX signal'],'SgnStartBit',0,'SgnLength',8,'SgnType',0,'ModeValue',-1,'DataType',0,'SLDataType','SS_DOUBLE','ByteLayout',0,'Factor',1,'Offset',0,'Min',0,'Max',255,'SgnComment',{{}},'SgnUnit',''),'MsgIdNumFormat',0,'MsgComment',{{''}}),'Version',1.2,'general',struct('isFromLib',1)),'GroupId',struct('Group',{{'RTICAN'}},'No',1,'Behavior',{{'NAMECHANGE'}},'BlockType',{{'SINK'}},'NameChangeFlag',0),'SFcnRTICANMessage',struct('MsgType','RX','MsgName',['RX Message'],'MsgIdFormat','STD','MsgId',100,'MsgLength',8,'NumSignals',1,'SampleTime',-1,'Signal',struct('SgnName',['RX signal'],'SgnStartBit',0,'SgnLength',8,'SgnType','standard','ModeValue',-1,'DataType',['unsigned int'],'ByteLayout',['little endian'],'SLDataType','SS_DOUBLE','Factor',1,'Offset',0),'StatusSelected','yes','TimeSelected','yes','DeltaTimeSelected','yes','BytePortSelected','no','MessageLengthSelected','no','EnablePortSelected','no','UserCoding',struct('Selected','no','InterfaceFile','UserDecodingFile','FcnName','UserDecodeFcn','InportSelected','no','InportWidth',1,'OutportSelected','no','OutportWidth',1),'TriggerPort',struct('Selected','no','TriggerType','rising'),'UseRXService','no','BoardType','DS4302','BoardNo',1,'ControllerNo',1,'SFcnPortType','Scalar'),'TLCFileName','rtican_rx_message')
      settings: AttributesFormatString=Group Id: RTICAN3\n
  SpeedControlEcho : rtican/RTICAN Receive (RX)   Reserved1=[]  Reserved2=[]  Reserved3=[]  Reserved4=[]  SfcnMessage=[]  Msg_Struct=[]  BoardTypeNo=[]  BoardNo=[]  ChannelNo=[]  Parameters=[]  DialogFcn=[]  UnitName=[]  Revision=[]  UnitValues=[]  DSProperties=struct('RTI',struct('Version',uint32(5),'BlockType',struct('isSLSource',uint8(1),'isSLSink',uint8(1),'isHWSource',uint8(0),'isHWSink',uint8(0),'isSetup',uint8(0),'isInline',uint8(1),'isNonInline',uint8(0),'isInterrupt',uint8(0),'isChannelwise',uint8(0)),'IOBoardType','RTICAN','UnitType','MESSAGE','Identifier','RX','DialogType','MSVC','BlockSet','RTICAN','SlaveProcessor','CAN'))  RTIBlockInterface=struct('OutputPortsWidth',int32([1 1 1 1 1 1]),'OutputPortsActive',[1 1 1 1 1 1],'OutputPortsName',{{'PID_DivisorEcho','D_NumeratorEcho','I_NumeratorEcho','P_NumeratorEcho',['RX status'],['RX time']}},'OutputPortsDataType',{{'SS_UINT16','SS_UINT16','SS_UINT16','SS_UINT16','SS_DOUBLE','SS_DOUBLE'}},'OutputPortsLabel',{{'PID_DivisorEcho','D_NumeratorEcho','I_NumeratorEcho','P_NumeratorEcho','',''}},'OutputPortsLabelMode','ON','InputPortsWidth',int32(0),'InputPortsActive',0,'DialogFcn','rtican_message_interface_gui','BlockDisplay',{{'','center'}},'IconTransparency','on','ParameterTunableNames',{{}},'InitLevel',3,'BlockName',struct('Token',{{'SpeedControlEcho'}}),'SampleTime',{{-1}},'TriggerPort',{{'none'}},'EnablePort',{{'none'}})  RTIBlockParameters=struct('BoardTypeNo',{{1,'OFF',[]}},'BoardNo',{{2,'ON',[1 16]}},'ChannelNo',{{1,'ON',[1 2]}},'Parameters',{{struct('DataFileSupport',struct('DataFileSelectedMaster',1,'DataFileSelectedLocal',1,'DataFileName','c:\users\leidos\development\carmaplatform\microautobox\src\data_files\srx_command.dbc|','DataFileDate',['17-Aug-2015 10:52:13'],'SelectedFile','..\data_files\srx_command.dbc','InterfaceFcn','rtican_dbc_file_parser'),'Options',struct('StatusSelected',1,'TimeSelected',1,'DeltaTimeSelected',0,'BytePortSelected',0,'MessageLengthSelected',0,'TriggerPort',struct('Selected',0,'TriggerType',0),'UserCoding',struct('Selected',0,'InterfaceFile','UserDecodingFile','FcnName','UserDecodeFcn','InportSelected',0,'InportWidth',1,'OutportSelected',0,'OutportWidth',1),'EnablePortSelected',0,'SignalOnPortnameSelected',1,'UseRXService',1),'Message',struct('MsgOnBlocknameSelected',1,'MsgName','SpeedControlEcho','MsgIdFormat',0,'MsgId',273,'MsgLength',8,'NumSignals',4,'SampleTime',-1,'Signal',struct('SgnName',{'PID_DivisorEcho','D_NumeratorEcho','I_NumeratorEcho','P_NumeratorEcho'},'SgnStartBit',{0,16,32,48},'SgnLength',{16,16,16,16},'ByteLayout',{2,2,2,2},'Factor',{1,1,1,1},'Offset',{0,0,0,0},'SgnComment',{'','','',''},'SgnUnit',{'','','',''},'Min',{0,0,0,0},'Max',{0,0,0,0},'SgnType',{0,0,0,0},'SLDataType',{'SS_UINT16','SS_UINT16','SS_UINT16','SS_UINT16'},'DataType',{0,0,0,0},'ModeValue',{-1,-1,-1,-1}),'MsgIdNumFormat',0,'MsgComment',{{''}}),'Version',1.2,'general',struct('isFromLib',0)),'OFF',[]}},'GroupId',{{struct('Group',{{'RTICAN'}},'No',3,'Behavior',{{'NAMECHANGE'}},'BlockType',{{'SINK'}},'NameChangeFlag',0),'OFF',[]}},'SFcnRTICANMessage',{{struct('MsgType','RX','SFcnPortType','Scalar','MsgName','SpeedControlEcho','MsgIdFormat','STD','MsgId',273,'MsgLength',8,'NumSignals',4,'SampleTime',-1,'Signal',struct('SgnName',{'PID_DivisorEcho','D_NumeratorEcho','I_NumeratorEcho','P_NumeratorEcho'},'SgnStartBit',{0,16,32,48},'SgnLength',{16,16,16,16},'ByteLayout',{['motorola back.'],['motorola back.'],['motorola back.'],['motorola back.']},'Factor',{1,1,1,1},'Offset',{0,0,0,0},'SgnType',{'standard','standard','standard','standard'},'SLDataType',{'SS_UINT16','SS_UINT16','SS_UINT16','SS_UINT16'},'DataType',{['unsigned int'],['unsigned int'],['unsigned int'],['unsigned int']},'ModeValue',{-1,-1,-1,-1}),'StatusSelected','yes','TimeSelected','yes','DeltaTimeSelected','no','BytePortSelected','no','MessageLengthSelected','no','TriggerPort',struct('Selected','no','TriggerType',0),'UserCoding',struct('Selected','no','InterfaceFile','UserDecodingFile','FcnName','UserDecodeFcn','InportSelected','no','InportWidth',1,'OutportSelected','no','OutportWidth',1),'EnablePortSelected','no','UseRXService','yes','BoardType','DS1','BoardNo',2,'ControllerNo',1),'OFF',[]}},'TLCFileName',{{'rtican_rx_message','OFF',[]}})  RTISFcnParameters=struct('SFcnRTICANMessage','struct','TLCFileName','char')  RTIBlockParaDefault=struct('BoardTypeNo',4302,'BoardNo',1,'ChannelNo',1,'Parameters',struct('DataFileSupport',struct('DataFileSelectedMaster',0,'DataFileSelectedLocal',0,'DataFileName','','DataFileDate','','SelectedFile',['<no file selected>']),'Options',struct('StatusSelected',1,'TimeSelected',1,'DeltaTimeSelected',1,'BytePortSelected',0,'MessageLengthSelected',0,'TriggerPort',struct('Selected',0,'TriggerType','rising'),'UserCoding',struct('Selected',0,'InterfaceFile','UserDecodingFile','FcnName','UserDecodeFcn','InportSelected',0,'InportWidth',1,'OutportSelected',0,'OutportWidth',1),'EnablePortSelected',0,'SignalOnPortnameSelected',1,'UseRXService',0),'Message',struct('MsgOnBlocknameSelected',0,'MsgName',['RX Message'],'MsgIdFormat',0,'MsgId',100,'MsgLength',8,'NumSignals',1,'SampleTime',-1,'Signal',struct('SgnName',['RX signal'],'SgnStartBit',0,'SgnLength',8,'SgnType',0,'ModeValue',-1,'DataType',0,'SLDataType','SS_DOUBLE','ByteLayout',0,'Factor',1,'Offset',0,'Min',0,'Max',255,'SgnComment',{{}},'SgnUnit',''),'MsgIdNumFormat',0,'MsgComment',{{''}}),'Version',1.2,'general',struct('isFromLib',1)),'GroupId',struct('Group',{{'RTICAN'}},'No',1,'Behavior',{{'NAMECHANGE'}},'BlockType',{{'SINK'}},'NameChangeFlag',0),'SFcnRTICANMessage',struct('MsgType','RX','MsgName',['RX Message'],'MsgIdFormat','STD','MsgId',100,'MsgLength',8,'NumSignals',1,'SampleTime',-1,'Signal',struct('SgnName',['RX signal'],'SgnStartBit',0,'SgnLength',8,'SgnType','standard','ModeValue',-1,'DataType',['unsigned int'],'ByteLayout',['little endian'],'SLDataType','SS_DOUBLE','Factor',1,'Offset',0),'StatusSelected','yes','TimeSelected','yes','DeltaTimeSelected','yes','BytePortSelected','no','MessageLengthSelected','no','EnablePortSelected','no','UserCoding',struct('Selected','no','InterfaceFile','UserDecodingFile','FcnName','UserDecodeFcn','InportSelected','no','InportWidth',1,'OutportSelected','no','OutportWidth',1),'TriggerPort',struct('Selected','no','TriggerType','rising'),'UseRXService','no','BoardType','DS4302','BoardNo',1,'ControllerNo',1,'SFcnPortType','Scalar'),'TLCFileName','rtican_rx_message')
      settings: AttributesFormatString=Group Id: RTICAN3\n
  UTC_Time : rtican/RTICAN Receive (RX)   Reserved1=[]  Reserved2=[]  Reserved3=[]  Reserved4=[]  SfcnMessage=[]  Msg_Struct=[]  BoardTypeNo=[]  BoardNo=[]  ChannelNo=[]  Parameters=[]  DialogFcn=[]  UnitName=[]  Revision=[]  UnitValues=[]  DSProperties=struct('RTI',struct('Version',uint32(5),'BlockType',struct('isSLSource',uint8(1),'isSLSink',uint8(1),'isHWSource',uint8(0),'isHWSink',uint8(0),'isSetup',uint8(0),'isInline',uint8(1),'isNonInline',uint8(0),'isInterrupt',uint8(0),'isChannelwise',uint8(0)),'IOBoardType','RTICAN','UnitType','MESSAGE','Identifier','RX','DialogType','MSVC','BlockSet','RTICAN','SlaveProcessor','CAN'))  RTIBlockInterface=struct('OutputPortsWidth',int32([1 1 1 1]),'OutputPortsActive',[1 1 1 1],'OutputPortsName',{{'UTC_Lower','UTC_Upper',['RX status'],['RX time']}},'OutputPortsDataType',{{'SS_UINT32','SS_UINT32','SS_DOUBLE','SS_DOUBLE'}},'OutputPortsLabel',{{'UTC_Lower','UTC_Upper','',''}},'OutputPortsLabelMode','ON','InputPortsWidth',int32(0),'InputPortsActive',0,'DialogFcn','rtican_message_interface_gui','BlockDisplay',{{'','center'}},'IconTransparency','on','ParameterTunableNames',{{}},'InitLevel',3,'BlockName',struct('Token',{{'UTC_Time'}}),'SampleTime',{{-1}},'TriggerPort',{{'none'}},'EnablePort',{{'none'}})  RTIBlockParameters=struct('BoardTypeNo',{{1,'OFF',[]}},'BoardNo',{{2,'ON',[1 16]}},'ChannelNo',{{1,'ON',[1 2]}},'Parameters',{{struct('DataFileSupport',struct('DataFileSelectedMaster',1,'DataFileSelectedLocal',1,'DataFileName','c:\users\leidos\development\carmaplatform\microautobox\src\data_files\srx_command.dbc|','DataFileDate',['17-Aug-2015 10:52:13'],'SelectedFile','..\data_files\srx_command.dbc','InterfaceFcn','rtican_dbc_file_parser'),'Options',struct('StatusSelected',1,'TimeSelected',1,'DeltaTimeSelected',0,'BytePortSelected',0,'MessageLengthSelected',0,'TriggerPort',struct('Selected',0,'TriggerType',0),'UserCoding',struct('Selected',0,'InterfaceFile','UserDecodingFile','FcnName','UserDecodeFcn','InportSelected',0,'InportWidth',1,'OutportSelected',0,'OutportWidth',1),'EnablePortSelected',0,'SignalOnPortnameSelected',1,'UseRXService',1),'Message',struct('MsgOnBlocknameSelected',1,'MsgName','UTC_Time','MsgIdFormat',0,'MsgId',90,'MsgLength',8,'NumSignals',2,'SampleTime',-1,'Signal',struct('SgnName',{'UTC_Lower','UTC_Upper'},'SgnStartBit',{0,32},'SgnLength',{32,32},'SgnType',{0,0},'ModeValue',{-1,-1},'DataType',{0,0},'ByteLayout',{2,2},'Factor',{1,1},'Offset',{0,0},'SgnComment',{{''},{''}},'SgnUnit',{'',''},'Min',{0,0},'Max',{0,0},'SLDataType',{'SS_UINT32','SS_UINT32'}),'MsgIdNumFormat',0,'MsgComment',{{''}}),'Version',1.2,'general',struct('isFromLib',0)),'OFF',[]}},'GroupId',{{struct('Group',{{'RTICAN'}},'No',3,'Behavior',{{'NAMECHANGE'}},'BlockType',{{'SINK'}},'NameChangeFlag',0),'OFF',[]}},'SFcnRTICANMessage',{{struct('MsgType','RX','SFcnPortType','Scalar','MsgName','UTC_Time','MsgIdFormat','STD','MsgId',90,'MsgLength',8,'NumSignals',2,'SampleTime',-1,'Signal',struct('SgnName',{'UTC_Lower','UTC_Upper'},'SgnStartBit',{0,32},'SgnLength',{32,32},'SgnType',{'standard','standard'},'ModeValue',{-1,-1},'DataType',{['unsigned int'],['unsigned int']},'ByteLayout',{['motorola back.'],['motorola back.']},'Factor',{1,1},'Offset',{0,0},'SLDataType',{'SS_UINT32','SS_UINT32'}),'StatusSelected','yes','TimeSelected','yes','DeltaTimeSelected','no','BytePortSelected','no','MessageLengthSelected','no','TriggerPort',struct('Selected','no','TriggerType',0),'UserCoding',struct('Selected','no','InterfaceFile','UserDecodingFile','FcnName','UserDecodeFcn','InportSelected','no','InportWidth',1,'OutportSelected','no','OutportWidth',1),'EnablePortSelected','no','UseRXService','yes','BoardType','DS1','BoardNo',2,'ControllerNo',1),'OFF',[]}},'TLCFileName',{{'rtican_rx_message','OFF',[]}})  RTISFcnParameters=struct('SFcnRTICANMessage','struct','TLCFileName','char')  RTIBlockParaDefault=struct('BoardTypeNo',4302,'BoardNo',1,'ChannelNo',1,'Parameters',struct('DataFileSupport',struct('DataFileSelectedMaster',0,'DataFileSelectedLocal',0,'DataFileName','','DataFileDate','','SelectedFile',['<no file selected>']),'Options',struct('StatusSelected',1,'TimeSelected',1,'DeltaTimeSelected',1,'BytePortSelected',0,'MessageLengthSelected',0,'TriggerPort',struct('Selected',0,'TriggerType','rising'),'UserCoding',struct('Selected',0,'InterfaceFile','UserDecodingFile','FcnName','UserDecodeFcn','InportSelected',0,'InportWidth',1,'OutportSelected',0,'OutportWidth',1),'EnablePortSelected',0,'SignalOnPortnameSelected',1,'UseRXService',0),'Message',struct('MsgOnBlocknameSelected',0,'MsgName',['RX Message'],'MsgIdFormat',0,'MsgId',100,'MsgLength',8,'NumSignals',1,'SampleTime',-1,'Signal',struct('SgnName',['RX signal'],'SgnStartBit',0,'SgnLength',8,'SgnType',0,'ModeValue',-1,'DataType',0,'SLDataType','SS_DOUBLE','ByteLayout',0,'Factor',1,'Offset',0,'Min',0,'Max',255,'SgnComment',{{}},'SgnUnit',''),'MsgIdNumFormat',0,'MsgComment',{{''}}),'Version',1.2,'general',struct('isFromLib',1)),'GroupId',struct('Group',{{'RTICAN'}},'No',1,'Behavior',{{'NAMECHANGE'}},'BlockType',{{'SINK'}},'NameChangeFlag',0),'SFcnRTICANMessage',struct('MsgType','RX','MsgName',['RX Message'],'MsgIdFormat','STD','MsgId',100,'MsgLength',8,'NumSignals',1,'SampleTime',-1,'Signal',struct('SgnName',['RX signal'],'SgnStartBit',0,'SgnLength',8,'SgnType','standard','ModeValue',-1,'DataType',['unsigned int'],'ByteLayout',['little endian'],'SLDataType','SS_DOUBLE','Factor',1,'Offset',0),'StatusSelected','yes','TimeSelected','yes','DeltaTimeSelected','yes','BytePortSelected','no','MessageLengthSelected','no','EnablePortSelected','no','UserCoding',struct('Selected','no','InterfaceFile','UserDecodingFile','FcnName','UserDecodeFcn','InportSelected','no','InportWidth',1,'OutportSelected','no','OutportWidth',1),'TriggerPort',struct('Selected','no','TriggerType','rising'),'UseRXService','no','BoardType','DS4302','BoardNo',1,'ControllerNo',1,'SFcnPortType','Scalar'),'TLCFileName','rtican_rx_message')
      settings: AttributesFormatString=Group Id: RTICAN3\n
  SRX Command Bus Data : Outport
  wires:
  AccelModuleFeedback/7 -> Bus Creator1/7  "AccelInjectionMsg"
  AccelModuleFeedback/8 -> Bus Creator1/8  "AccelPairTimeoutFlag"
  AccelModuleFeedback/2 -> Bus Creator1/2  "AccelCmdInjectionFlag"
  AccelModuleFeedback/6 -> Bus Creator1/6  "AccelDriverOverride"
  AccelModuleFeedback/5 -> Bus Creator1/5  "AccelCanTimeoutFlag"
  AccelModuleFeedback/4 -> Bus Creator1/4  "AccelCmdModeEcho"
  AccelModuleFeedback/1 -> Bus Creator1/1  "Torque"
  AccelModuleFeedback/3 -> Bus Creator1/3  "AccelCmdTimeoutFlag"
  AccelModuleFeedback/10 -> Bus Creator1/10  "time"
  AccelModuleFeedback/9 -> Bus Creator1/9  "status"
  BrakeModuleFeedback/8 -> Bus Creator2/8  "BrakePairTimeoutFlag"
  BrakeModuleFeedback/6 -> Bus Creator2/6  "BrakeDriverOverride"
  BrakeModuleFeedback/2 -> Bus Creator2/2  "BrakeCmdInjectionFlag"
  BrakeModuleFeedback/4 -> Bus Creator2/4  "BrakeCmdModeEcho"
  BrakeModuleFeedback/3 -> Bus Creator2/3  "BrakeCmdTimeoutFlag"
  BrakeModuleFeedback/5 -> Bus Creator2/5  "BrakeCanTimoutFlag"
  BrakeModuleFeedback/7 -> Bus Creator2/7  "BrakeInjectionMsg"
  BrakeModuleFeedback/1 -> Bus Creator2/1  "BrakeForce"
  BrakeModuleFeedback/9 -> Bus Creator2/9  "status"
  BrakeModuleFeedback/10 -> Bus Creator2/10  "time"
  FrontLightStatus/2 -> Bus Creator3/2  "FrontOutput2"
  FrontLightStatus/5 -> Bus Creator3/5  "FrontOutput5"
  FrontLightStatus/3 -> Bus Creator3/3  "FrontOutput3"
  FrontLightStatus/6 -> Bus Creator3/6  "FrontOutput6"
  FrontLightStatus/4 -> Bus Creator3/4  "FrontOutput4"
  FrontLightStatus/1 -> Bus Creator3/1  "FrontOutput1"
  FrontLightStatus/7 -> Bus Creator3/7  "status"
  FrontLightStatus/8 -> Bus Creator3/8  "time"
  RearLightStatus/7 -> Bus Creator4/7  "status"
  RearLightStatus/8 -> Bus Creator4/8  "time"
  RearLightStatus/1 -> Bus Creator4/1  "RearOutput1"
  RearLightStatus/2 -> Bus Creator4/2  "RearOutput2"
  RearLightStatus/6 -> Bus Creator4/6  "RearOutput6"
  RearLightStatus/3 -> Bus Creator4/3  "RearOutput3"
  RearLightStatus/4 -> Bus Creator4/4  "RearOutput4"
  RearLightStatus/5 -> Bus Creator4/5  "RearOutput5"
  SpeedControlEcho/4 -> Bus Creator5/4  "P_NumeratorEcho"
  SpeedControlEcho/3 -> Bus Creator5/3  "I_NumeratorEcho"
  SpeedControlEcho/1 -> Bus Creator5/1  "PID_DivisorEcho"
  SpeedControlEcho/2 -> Bus Creator5/2  "D_NumeratorEcho"
  SpeedControlEcho/5 -> Bus Creator5/5  "status"
  SpeedControlEcho/6 -> Bus Creator5/6  "time"
  Bus Creator/1 -> Bus Creator6/1  "UTC Time"
  Bus Creator1/1 -> Bus Creator6/2  "Accel Module Feedback"
  Bus Creator2/1 -> Bus Creator6/3  "Brake Module Feedback"
  Bus Creator3/1 -> Bus Creator6/4  "Front Light Status"
  Bus Creator4/1 -> Bus Creator6/5  "Rear Light Status"
  Bus Creator5/1 -> Bus Creator6/6  "Speed Control Echo"
  Bus Creator6/1 -> SRX Command Bus Data/1
  UTC_Time/2 -> Bus Creator/2  "UTC_Upper"
  UTC_Time/1 -> Bus Creator/1  "UTC_Lower"
  UTC_Time/3 -> Bus Creator/3  "status"
  UTC_Time/4 -> Bus Creator/4  "time"

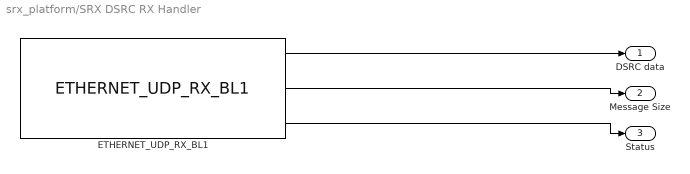
== system srx_platform/SRX DSRC RX Handler ==
  ETHERNET_UDP_RX_BL1 : rtiethernetudplib/ETHERNET_UDP_RX_BL1  InterfaceName=rti_ethernet_interface_name  BoardType=ETH Type 1  ModuleNo=1  ChannelNo=1  SocketNo=2  MaxMessageSize=1472  LocalSocket=192.168.88.21:5001  RemoteSocket=192.168.88.10:5001  DSProperties=struct('RTI',struct('Version',uint32(1),'BlockType',struct('isSLSource',uint8(1),'isSLSink',uint8(0),'isHWSource',uint8(0),'isHWSink',uint8(1),'isSetup',uint8(0),'isInline',uint8(1),'isNonInline',uint8(1),'isInterrupt',uint8(0),'isChannelwise',uint8(1)),'IOBoardType','DSETHERNETUDP','UnitType','ETHUDP','Identifier','RX','DialogType','SL','BlockSet','RTIETHERNETUDP','SlaveProcessor','NONE'))  RTIBlockInterface=struct('OutputPortsWidth',int32([1 1 1]),'OutputPortsActive',[1 1 1],'OutputPortsName',{{'Data',['Message Size'],'Status'}},'OutputPortsDataType',{{'SS_UINT32','SS_INT32','SS_BOOLEAN'}},'BlockDisplay',{{['Ethernet UDP Receive\nBoard Type: ETH Type 1\nModule: 1\nSocket: 2\nMaximum Message Size: 1472'],'center'}},'IconTransparency','on','InitLevel',3,'BlockName',struct('Token',{{'ETHERNET_UDP_RX_BL1'}}),'MaskDescription',['To receive messages from the Ethernet UDP interface.'])  RTIBlockParameters=struct('InterfaceName',{{'rti_ethernet_interface_name','OFF',[]}},'BoardType',{{1,'OFF',[]}},'ModuleNo',{{1,'OFF',[1 16]}},'ChannelNo',{{1,'OFF',[1 2]}},'SocketNo',{{2,'OFF',[1 4]}},'MaxMessageSize',{{1472,'ON',[1 1472]}},'LocalSocket',{{'192.168.88.21:5001','OFF',[]}},'RemoteSocket',{{'192.168.88.10:5001','OFF',[]}})  RTISFcnParameters=struct('InterfaceName','char','BoardType','double','ModuleNo','double','ChannelNo','double','SocketNo','double','MaxMessageSize','double','LocalSocket','char','RemoteSocket','char')  RTIBlockParaDefault=struct('InterfaceName','rti_ethernet_interface_name','BoardType',1,'ModuleNo',1,'ChannelNo',1,'SocketNo',1,'MaxMessageSize',625,'LocalSocket','XXX.XXX.XXX.XXX:5000','RemoteSocket','XXX.XXX.XXX.XXX:5000')
  DSRC data : Outport
  Message Size : Outport  Port=2
  Status : Outport  Port=3
  wires:
  ETHERNET_UDP_RX_BL1/1 -> DSRC data/1
  ETHERNET_UDP_RX_BL1/2 -> Message Size/1
  ETHERNET_UDP_RX_BL1/3 -> Status/1

== system srx_platform/SRX HMI UDP RX Handler ==
  note: TODO: parse out requested CACC state
      | from udp message and set in GlobalStoreBus
  ETHERNET_UDP_RX_BL1 : rtiethernetudplib/ETHERNET_UDP_RX_BL1  InterfaceName=rti_ethernet_interface_name  BoardType=ETH Type 1  ModuleNo=1  ChannelNo=1  SocketNo=4  MaxMessageSize=625  LocalSocket=192.168.88.21:47356  RemoteSocket=192.168.88.169:47357  DSProperties=struct('RTI',struct('Version',uint32(1),'BlockType',struct('isSLSource',uint8(1),'isSLSink',uint8(0),'isHWSource',uint8(0),'isHWSink',uint8(1),'isSetup',uint8(0),'isInline',uint8(1),'isNonInline',uint8(1),'isInterrupt',uint8(0),'isChannelwise',uint8(1)),'IOBoardType','DSETHERNETUDP','UnitType','ETHUDP','Identifier','RX','DialogType','SL','BlockSet','RTIETHERNETUDP','SlaveProcessor','NONE'))  RTIBlockInterface=struct('OutputPortsWidth',int32([1 1 1]),'OutputPortsActive',[1 1 1],'OutputPortsName',{{'Data',['Message Size'],'Status'}},'OutputPortsDataType',{{'SS_UINT32','SS_INT32','SS_BOOLEAN'}},'BlockDisplay',{{['Ethernet UDP Receive\nBoard Type: ETH Type 1\nModule: 1\nSocket: 4\nMaximum Message Size: 625'],'center'}},'IconTransparency','on','InitLevel',3,'BlockName',struct('Token',{{'ETHERNET_UDP_RX_BL1'}}),'MaskDescription',['To receive messages from the Ethernet UDP interface.'])  RTIBlockParameters=struct('InterfaceName',{{'rti_ethernet_interface_name','OFF',[]}},'BoardType',{{1,'OFF',[]}},'ModuleNo',{{1,'OFF',[1 16]}},'ChannelNo',{{1,'OFF',[1 2]}},'SocketNo',{{4,'OFF',[1 4]}},'MaxMessageSize',{{625,'ON',[1 1472]}},'LocalSocket',{{'192.168.88.21:47356','OFF',[]}},'RemoteSocket',{{'192.168.88.169:47357','OFF',[]}})  RTISFcnParameters=struct('InterfaceName','char','BoardType','double','ModuleNo','double','ChannelNo','double','SocketNo','double','MaxMessageSize','double','LocalSocket','char','RemoteSocket','char')  RTIBlockParaDefault=struct('InterfaceName','rti_ethernet_interface_name','BoardType',1,'ModuleNo',1,'ChannelNo',1,'SocketNo',1,'MaxMessageSize',625,'LocalSocket','XXX.XXX.XXX.XXX:5000','RemoteSocket','XXX.XXX.XXX.XXX:5000')
  HMI Data : Outport
  wires:
  ETHERNET_UDP_RX_BL1/2 -> ?
  ETHERNET_UDP_RX_BL1/3 -> ?
  ETHERNET_UDP_RX_BL1/1 -> ?
  ? -> HMI Data/1
